simulink model "feedbackLinearizationMambo"  (R2021a)
settings: Solver=VariableStepAuto  StartTime=0.0  StopTime=10  FixedStep=4e-3  RelTol=1e-12
InitFcn:
  | init
values from neighbouring files (symbols this model uses):
  a = 4.7200e-08*13840.8    (= 0.00065328576)    [init.m]
  c = 1.1393e-10*13840.8    (= 1.576882344e-06)    [init.m]
  g = 9.31    [init.m]
  isMambo = true    [init.m]
  J = [Jx;Jy;Jz]    [init.m]
  Jx = 5.82857e-5    (= 5.82857e-05)    [init.m]
  Jy = 7.169148e-5    (= 7.169148e-05)    [init.m]
  Jz = 1e-4    (= 0.0001)    [init.m]
  Ki = [0.1 0.6 0.1]*0    [init.m]
  Kp = [0.6 0.7 1]*50    [init.m]
  Kw = [0.08 0.1 0.2]*100    [init.m]
  l = 0.0624*2    (= 0.1248)    [init.m]
  m = 0.063    [init.m]
  posNED = [57 95 -0.046]    [init.m]
  sigma = [l*a/Jx l*a/Jy l*a/Jz a/m]    [init.m]
  T = 0.0050    (= 0.005)    [init.m]
undefined symbols (not defined in the file or in its folder): DiscIntNeverNeededParam, Earth, init, rho, Vehicle, WGS84
libraries: pid_lib x14, sharedtransform x6, simulink x2, shared6dof x1, aerolibasang x1, aerolibtransform2 x1, vrlib x1
(part 1 of 2)
settings Model: Creator=dbnun  LastModifiedBy=dbnun
settings SolverCC: AlgebraicLoopSolver=TrustRegion

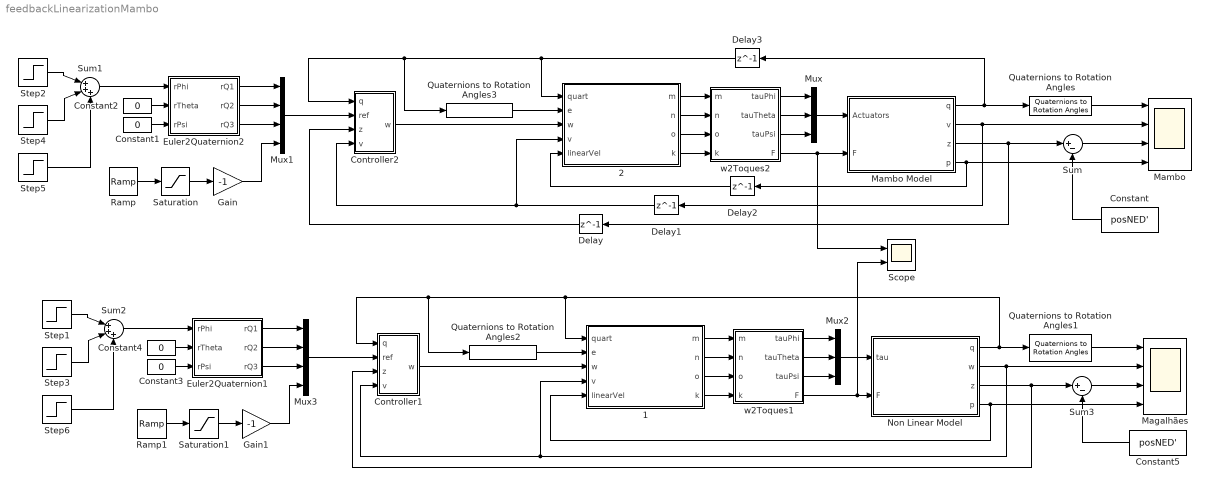
== system feedbackLinearizationMambo ==
  " 1" : MATLAB Function  TreatAsAtomicUnit=on
  " 2" : MATLAB Function  TreatAsAtomicUnit=on
  Constant : Constant  Value=posNED'
  Constant{1..4} (4 alike) : Constant  Value=0
  Constant5 : Constant  Value=posNED'
  Controller1 : Subsystem
  Controller2 : Subsystem
  Delay : Delay  DelayLength=1  InitialCondition=posNED'
  Delay1 : Delay  DelayLength=1
  Delay2 : Delay  DelayLength=1
  Delay3 : Delay  DelayLength=1  InitialCondition=[1 0 0 0]
  Euler2Quaternion1 : Subsystem
  Euler2Quaternion2 : Subsystem
  Gain : Gain  Gain=-1
  Gain1 : Gain  Gain=-1
  Magalhães : Scope  NumInputPorts=4
  Mambo : Scope  NumInputPorts=4
  Mambo Model : Subsystem
  Mux : Mux  Inputs=3
  Mux1 : Mux
  Mux2 : Mux  Inputs=3
  Mux3 : Mux
  Non Linear Model : Subsystem
  Quaternions to Rotation Angles{,1..3} (4 alike) : sharedtransform/Quaternions to Rotation Angles  rotationOrder=XYZ  aMode=aMode
      settings: SourceProductBaseCode=AE,PW,DR,MT,UV,VE
  Ramp : simulink/Sources/Ramp  slope=2  start=0  InitialOutput=0
  Ramp1 : simulink/Sources/Ramp  slope=2  start=0  InitialOutput=0
  Saturation : Saturate  UpperLimit=1  LowerLimit=0
  Saturation1 : Saturate  UpperLimit=1  LowerLimit=0
  Scope : Scope  NumInputPorts=2
  Step1 : Step  Time=2  After=2*pi/180  SampleTime=0
  Step2 : Step  Time=2  After=2*pi/180  SampleTime=0
  Step3 : Step  Time=3  After=-3*pi/180  SampleTime=0
  Step4 : Step  Time=3  After=-3*pi/180  SampleTime=0
  Step5 : Step  Time=3.5  After=1*pi/180  SampleTime=0
  Step6 : Step  Time=3.5  After=1*pi/180  SampleTime=0
  Sum : Sum  Inputs=|+-
  Sum1 : Sum  Inputs=|+++
  Sum2 : Sum  Inputs=|+++
  Sum3 : Sum  Inputs=|+-
  w2Toques1 : Subsystem
  w2Toques2 : Subsystem
  wires:
  Mux/1 -> Mambo Model/1(Actuators)
  w2Toques2/1(tauPhi) -> Mux/1
  w2Toques2/2(tauTheta) -> Mux/2
  w2Toques2/3(tauPsi) -> Mux/3
  Quaternions to Rotation Angles/1 -> Mambo/1
  Quaternions to Rotation Angles1/1 -> Magalhães/1
  w2Toques1/3(tauPsi) -> Mux2/3
  Mux3/1 -> Controller1/2(ref)
  Non Linear Model/1(q) -> Quaternions to Rotation Angles2/1, Controller1/1(q), " 1"/1(quart), Quaternions to Rotation Angles1/1
  w2Toques1/1(tauPhi) -> Mux2/1
  " 1"/3(o) -> w2Toques1/3(o)
  Euler2Quaternion1/1(rQ1) -> Mux3/1
  " 1"/1(m) -> w2Toques1/1(m)
  Non Linear Model/2(w) -> Magalhães/2, " 1"/4(v), Controller1/4(v)
  " 1"/2(n) -> w2Toques1/2(n)
  w2Toques1/2(tauTheta) -> Mux2/2
  Euler2Quaternion1/2(rQ2) -> Mux3/2
  Euler2Quaternion1/3(rQ3) -> Mux3/3
  " 1"/4(k) -> w2Toques1/4(k)
  Non Linear Model/4(p) -> Magalhães/4, " 1"/5(linearVel)
  Non Linear Model/3(z) -> Sum3/1, Controller1/3(z)
  Mux2/1 -> Non Linear Model/1(tau)
  Controller1/1(w) -> " 1"/3(w)
  Quaternions to Rotation Angles2/1 -> " 1"/2(e)
  Constant1/1 -> Euler2Quaternion2/3(rPsi)
  Constant2/1 -> Euler2Quaternion2/2(rTheta)
  Controller2/1(w) -> " 2"/3(w)
  Euler2Quaternion2/2(rQ2) -> Mux1/2
  " 2"/2(n) -> w2Toques2/2(n)
  " 2"/3(o) -> w2Toques2/3(o)
  Euler2Quaternion2/1(rQ1) -> Mux1/1
  Mambo Model/2(v) -> Delay1/1, Mambo/2
  Mambo Model/1(q) -> Delay3/1, Quaternions to Rotation Angles/1
  Mambo Model/4(p) -> Mambo/4, Delay2/1
  Sum1/1 -> Euler2Quaternion2/1(rPhi)
  Mux1/1 -> Controller2/2(ref)
  Step5/1 -> Sum1/3
  Step4/1 -> Sum1/2
  " 2"/1(m) -> w2Toques2/1(m)
  Quaternions to Rotation Angles3/1 -> " 2"/2(e)
  Euler2Quaternion2/3(rQ3) -> Mux1/3
  Step2/1 -> Sum1/1
  Mambo Model/3(z) -> Sum/1, Delay/1
  w2Toques2/4(F) -> Scope/1, Mambo Model/2(F)
  " 2"/4(k) -> w2Toques2/4(k)
  Delay/1 -> Controller2/3(z)
  Delay1/1 -> " 2"/4(v), Controller2/4(v)
  Delay2/1 -> " 2"/5(linearVel)
  Delay3/1 -> " 2"/1(quart), Controller2/1(q), Quaternions to Rotation Angles3/1
  w2Toques1/4(F) -> Scope/2, Non Linear Model/2(F)
  Step6/1 -> Sum2/3
  Sum2/1 -> Euler2Quaternion1/1(rPhi)
  Step3/1 -> Sum2/2
  Step1/1 -> Sum2/1
  Constant4/1 -> Euler2Quaternion1/2(rTheta)
  Constant3/1 -> Euler2Quaternion1/3(rPsi)
  Sum/1 -> Mambo/3
  Sum3/1 -> Magalhães/3
  Constant/1 -> Sum/2
  Constant5/1 -> Sum3/2
  Saturation/1 -> Gain/1
  Ramp/1 -> Saturation/1
  Gain/1 -> Mux1/4
  Gain1/1 -> Mux3/4
  Saturation1/1 -> Gain1/1
  Ramp1/1 -> Saturation1/1

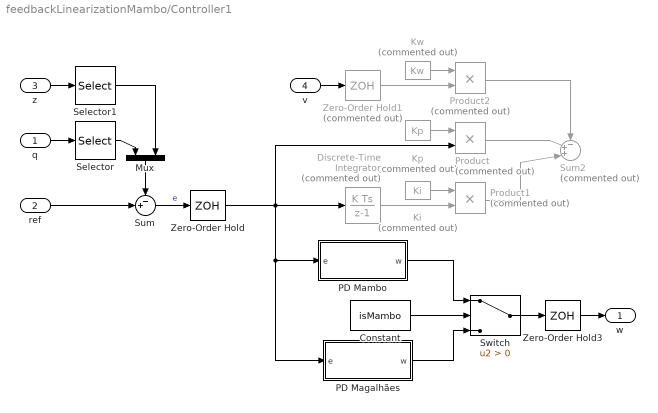
== system feedbackLinearizationMambo/Controller1 ==
  q : Inport
  ref : Inport  Port=2
  z : Inport  Port=3
  v : Inport  Port=4
  Constant : Constant  Value=isMambo
  Discrete-Time Integrator : DiscreteIntegrator  Commented=on  SampleTime=T  ICPrevOutput=DiscIntNeverNeededParam  ICPrevScaledInput=DiscIntNeverNeededParam
  Ki : Constant  Commented=on  Value=Ki
  Kp : Constant  Commented=on  Value=Kp
  Kw : Constant  Commented=on  Value=Kw  VectorParams1D=off
  Mux : Mux  Inputs=2
  PD Magalhães : Subsystem
  PD Mambo : Subsystem
  Product : Product  Commented=on
  Product1 : Product  Commented=on
  Product2 : Product  Commented=on
  Selector : Selector  InputPortWidth=4  IndexOptions=Index vector (dialog)  Indices=[2 3 4]  OutputSizes=1
  Selector1 : Selector  InputPortWidth=3  IndexOptions=Index vector (dialog)  Indices=[3]  OutputSizes=1
  Sum : Sum  Inputs=-+|
  Sum2 : Sum  Commented=on  Inputs=-++|
  Switch : Switch  Criteria=u2 > Threshold
  Zero-Order Hold : ZeroOrderHold  SampleTime=T
  Zero-Order Hold1 : ZeroOrderHold  Commented=on  SampleTime=T
  Zero-Order Hold3 : ZeroOrderHold  SampleTime=T
  w : Outport
  wires:
  Ki/1 -> Product1/1
  Selector/1 -> Mux/1
  q/1 -> Selector/1
  Product1/1 -> Sum2/3
  Sum/1 -> Zero-Order Hold/1  "e"
  ref/1 -> Sum/2
  Kw/1 -> Product2/1
  Product/1 -> Sum2/2
  Product2/1 -> Sum2/1
  Kp/1 -> Product/1
  v/1 -> Zero-Order Hold1/1
  Discrete-Time Integrator/1 -> Product1/2
  Zero-Order Hold/1 -> PD Magalhães/1(e), PD Mambo/1(e), Product/2, Discrete-Time Integrator/1
  Zero-Order Hold1/1 -> Product2/2
  PD Mambo/1(w) -> Switch/1
  Constant/1 -> Switch/2
  PD Magalhães/1(w) -> Switch/3
  Switch/1 -> Zero-Order Hold3/1
  Zero-Order Hold3/1 -> w/1
  z/1 -> Selector1/1
  Mux/1 -> Sum/1
  Selector1/1 -> Mux/2

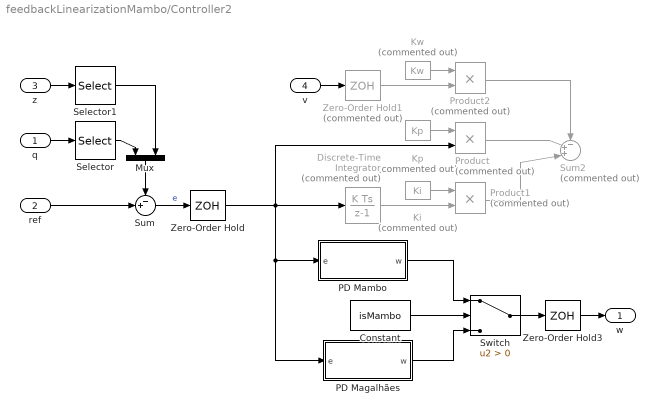
== system feedbackLinearizationMambo/Controller2 ==
  q : Inport
  ref : Inport  Port=2
  z : Inport  Port=3
  v : Inport  Port=4
  Constant : Constant  Value=isMambo
  Discrete-Time Integrator : DiscreteIntegrator  Commented=on  SampleTime=T  ICPrevOutput=DiscIntNeverNeededParam  ICPrevScaledInput=DiscIntNeverNeededParam
  Ki : Constant  Commented=on  Value=Ki
  Kp : Constant  Commented=on  Value=Kp
  Kw : Constant  Commented=on  Value=Kw  VectorParams1D=off
  Mux : Mux  Inputs=2
  PD Magalhães : Subsystem
  PD Mambo : Subsystem
  Product : Product  Commented=on
  Product1 : Product  Commented=on
  Product2 : Product  Commented=on
  Selector : Selector  InputPortWidth=4  IndexOptions=Index vector (dialog)  Indices=[2 3 4]  OutputSizes=1
  Selector1 : Selector  InputPortWidth=3  IndexOptions=Index vector (dialog)  Indices=[3]  OutputSizes=1
  Sum : Sum  Inputs=-+|
  Sum2 : Sum  Commented=on  Inputs=-++|
  Switch : Switch  Criteria=u2 > Threshold
  Zero-Order Hold : ZeroOrderHold  SampleTime=T
  Zero-Order Hold1 : ZeroOrderHold  Commented=on  SampleTime=T
  Zero-Order Hold3 : ZeroOrderHold  SampleTime=T
  w : Outport
  wires:
  Ki/1 -> Product1/1
  Selector/1 -> Mux/1
  q/1 -> Selector/1
  Product1/1 -> Sum2/3
  Sum/1 -> Zero-Order Hold/1  "e"
  ref/1 -> Sum/2
  Kw/1 -> Product2/1
  Product/1 -> Sum2/2
  Product2/1 -> Sum2/1
  Kp/1 -> Product/1
  v/1 -> Zero-Order Hold1/1
  Discrete-Time Integrator/1 -> Product1/2
  Zero-Order Hold/1 -> PD Magalhães/1(e), PD Mambo/1(e), Product/2, Discrete-Time Integrator/1
  Zero-Order Hold1/1 -> Product2/2
  PD Mambo/1(w) -> Switch/1
  Constant/1 -> Switch/2
  PD Magalhães/1(w) -> Switch/3
  Switch/1 -> Zero-Order Hold3/1
  Zero-Order Hold3/1 -> w/1
  z/1 -> Selector1/1
  Mux/1 -> Sum/1
  Selector1/1 -> Mux/2

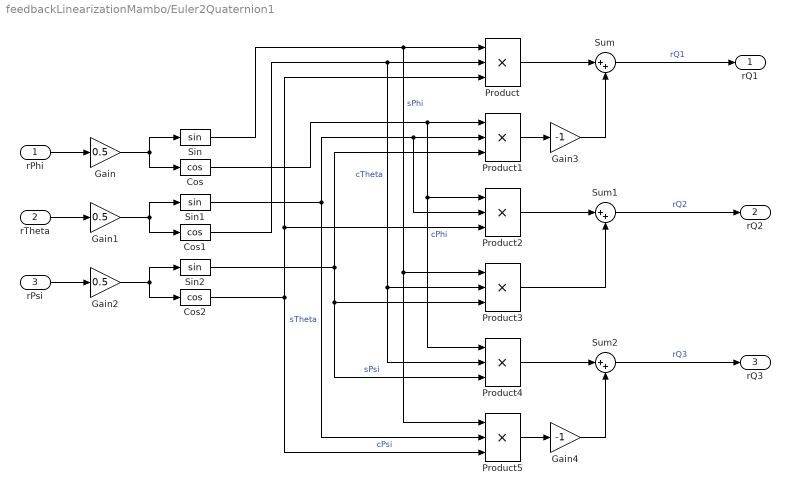
== system feedbackLinearizationMambo/Euler2Quaternion1 ==
  rPhi : Inport
  rTheta : Inport  Port=2
  rPsi : Inport  Port=3
  Cos : Trigonometry  Operator=cos
  Cos1 : Trigonometry  Operator=cos
  Cos2 : Trigonometry  Operator=cos
  Gain : Gain  Gain=0.5
  Gain1 : Gain  Gain=0.5
  Gain2 : Gain  Gain=0.5
  Gain3 : Gain  Gain=-1
  Gain4 : Gain  Gain=-1
  Product{,1..5} (6 alike) : Product  Inputs=3
  Sin : Trigonometry
  Sin1 : Trigonometry
  Sin2 : Trigonometry
  Sum : Sum  Inputs=|++
  Sum1 : Sum  Inputs=|++
  Sum2 : Sum  Inputs=|++
  rQ1 : Outport
  rQ2 : Outport  Port=2
  rQ3 : Outport  Port=3
  wires:
  Sum1/1 -> rQ2/1  "rQ2"
  rTheta/1 -> Gain1/1
  Gain/1 -> Sin/1, Cos/1
  rPsi/1 -> Gain2/1
  Sin1/1 -> Product2/2, Product1/2, Product5/2  "sTheta"
  Gain2/1 -> Sin2/1, Cos2/1
  rPhi/1 -> Gain/1
  Gain1/1 -> Sin1/1, Cos1/1
  Sin2/1 -> Product4/3, Product3/3, Product1/3  "sPsi"
  Cos/1 -> Product4/1, Product2/1, Product1/1  "cPhi"
  Sum2/1 -> rQ3/1  "rQ3"
  Cos2/1 -> Product2/3, Product/3, Product5/3  "cPsi"
  Sin/1 -> Product5/1, Product3/1, Product/1  "sPhi"
  Gain3/1 -> Sum/2
  Cos1/1 -> Product4/2, Product3/2, Product/2  "cTheta"
  Product1/1 -> Gain3/1
  Product/1 -> Sum/1
  Product5/1 -> Gain4/1
  Product3/1 -> Sum1/2
  Product2/1 -> Sum1/1
  Product4/1 -> Sum2/1
  Gain4/1 -> Sum2/2
  Sum/1 -> rQ1/1  "rQ1"

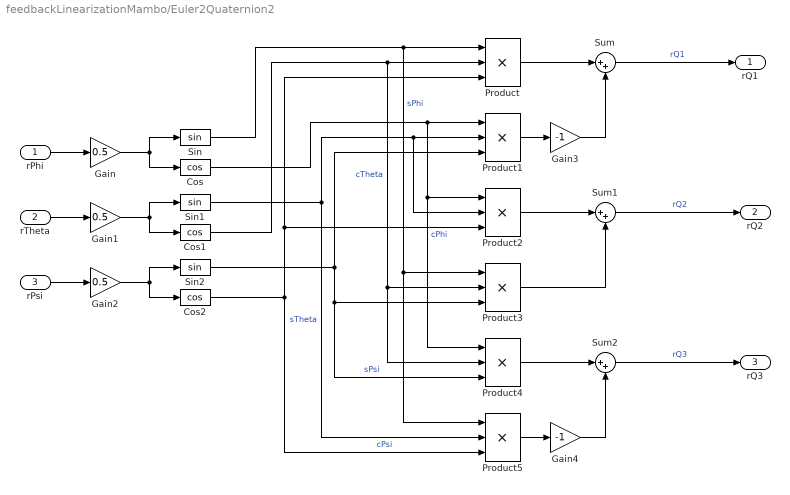
== system feedbackLinearizationMambo/Euler2Quaternion2 ==
  rPhi : Inport
  rTheta : Inport  Port=2
  rPsi : Inport  Port=3
  Cos : Trigonometry  Operator=cos
  Cos1 : Trigonometry  Operator=cos
  Cos2 : Trigonometry  Operator=cos
  Gain : Gain  Gain=0.5
  Gain1 : Gain  Gain=0.5
  Gain2 : Gain  Gain=0.5
  Gain3 : Gain  Gain=-1
  Gain4 : Gain  Gain=-1
  Product{,1..5} (6 alike) : Product  Inputs=3
  Sin : Trigonometry
  Sin1 : Trigonometry
  Sin2 : Trigonometry
  Sum : Sum  Inputs=|++
  Sum1 : Sum  Inputs=|++
  Sum2 : Sum  Inputs=|++
  rQ1 : Outport
  rQ2 : Outport  Port=2
  rQ3 : Outport  Port=3
  wires:
  Sum1/1 -> rQ2/1  "rQ2"
  rTheta/1 -> Gain1/1
  Gain/1 -> Sin/1, Cos/1
  rPsi/1 -> Gain2/1
  Sin1/1 -> Product2/2, Product1/2, Product5/2  "sTheta"
  Gain2/1 -> Sin2/1, Cos2/1
  rPhi/1 -> Gain/1
  Gain1/1 -> Sin1/1, Cos1/1
  Sin2/1 -> Product4/3, Product3/3, Product1/3  "sPsi"
  Cos/1 -> Product4/1, Product2/1, Product1/1  "cPhi"
  Sum2/1 -> rQ3/1  "rQ3"
  Cos2/1 -> Product2/3, Product/3, Product5/3  "cPsi"
  Sin/1 -> Product5/1, Product3/1, Product/1  "sPhi"
  Gain3/1 -> Sum/2
  Cos1/1 -> Product4/2, Product3/2, Product/2  "cTheta"
  Product1/1 -> Gain3/1
  Product/1 -> Sum/1
  Product5/1 -> Gain4/1
  Product3/1 -> Sum1/2
  Product2/1 -> Sum1/1
  Product4/1 -> Sum2/1
  Gain4/1 -> Sum2/2
  Sum/1 -> rQ1/1  "rQ1"

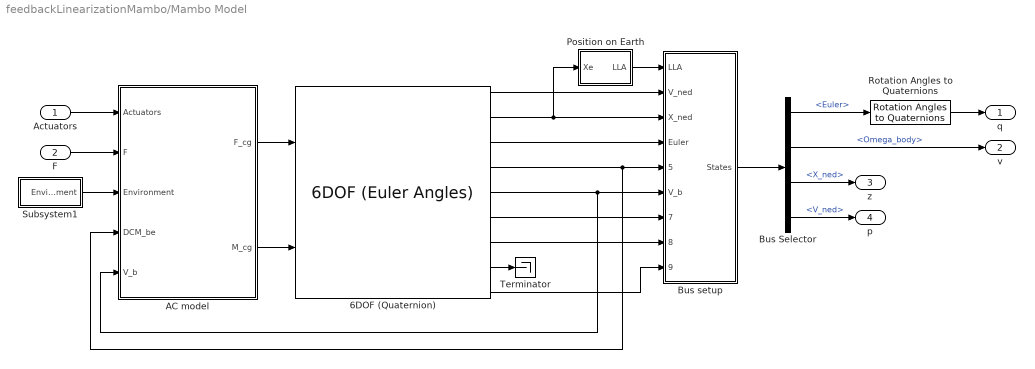
== system feedbackLinearizationMambo/Mambo Model ==
  Actuators : Inport
  F : Inport  Port=2
  6DOF (Quaternion) : shared6dof/6DOF (Euler Angles)  units=Metric (MKS)  mtype=Fixed  rep=Euler Angles  xme_0=init.posNED  Vm_0=init.vb  eul_0=init.euler  pm_0=init.angRates  mass_0=Vehicle.Airframe.mass  mass_e=0.5  mass_f=2.0  inertia=Vehicle.Airframe.inertia  inertia_e=eye(3)  inertia_f=2*eye(3)  k_quat=Vehicle.SixDOF.quatGain  vre_flag=on  abi_flag=on  aMode=aMode  xme_statename=''  Vm_statename=''  eul_statename=''  quat_statename=''  pm_statename=''  mass_statename=''
      settings: SourceProductBaseCode=AE,PW,DR,MT,UV,VE
  AC model : Subsystem
  Bus Selector : BusSelector  OutputSignals=Euler,Omega_body,X_ned,V_ned
  Bus setup : Subsystem
  Position on Earth : Subsystem  Priority=1  TreatAsAtomicUnit=on
  Rotation Angles to Quaternions : sharedtransform/Rotation Angles to Quaternions  rotationOrder=XYZ  aMode=aMode
      settings: SourceProductBaseCode=AE,PW,DR,MT,UV,VE
  Subsystem1 : Subsystem
  Terminator : Terminator
  q : Outport
  v : Outport  Port=2
  z : Outport  Port=3
  p : Outport  Port=4
  wires:
  Position on Earth/1(LLA) -> Bus setup/1(LLA)
  6DOF (Quaternion)/5 -> AC model/5(V_b), Bus setup/6(V_b)
  6DOF (Quaternion)/7 -> Bus setup/8(dOmega_b)
  Subsystem1/1(Environment) -> AC model/3(Environment)
  6DOF (Quaternion)/1 -> Bus setup/2(V_ned)
  6DOF (Quaternion)/8 -> Terminator/1
  Bus setup/1(States) -> Bus Selector/1
  AC model/1(F_cg) -> 6DOF (Quaternion)/1
  6DOF (Quaternion)/6 -> Bus setup/7(Omega_b)
  6DOF (Quaternion)/2 -> Position on Earth/1(Xe), Bus setup/3(X_ned)
  6DOF (Quaternion)/3 -> Bus setup/4(Euler)
  Actuators/1 -> AC model/1(Actuators)
  6DOF (Quaternion)/9 -> Bus setup/9(Accel_b)
  AC model/2(M_cg) -> 6DOF (Quaternion)/2
  6DOF (Quaternion)/4 -> AC model/4(DCM_be), Bus setup/5(DCM_be)
  Bus Selector/1 -> Rotation Angles to Quaternions/1  "<Euler>"
  Rotation Angles to Quaternions/1 -> q/1
  Bus Selector/2 -> v/1  "<Omega_body>"
  Bus Selector/3 -> z/1  "<X_ned>"
  Bus Selector/4 -> p/1  "<V_ned>"
  F/1 -> AC model/2(F)

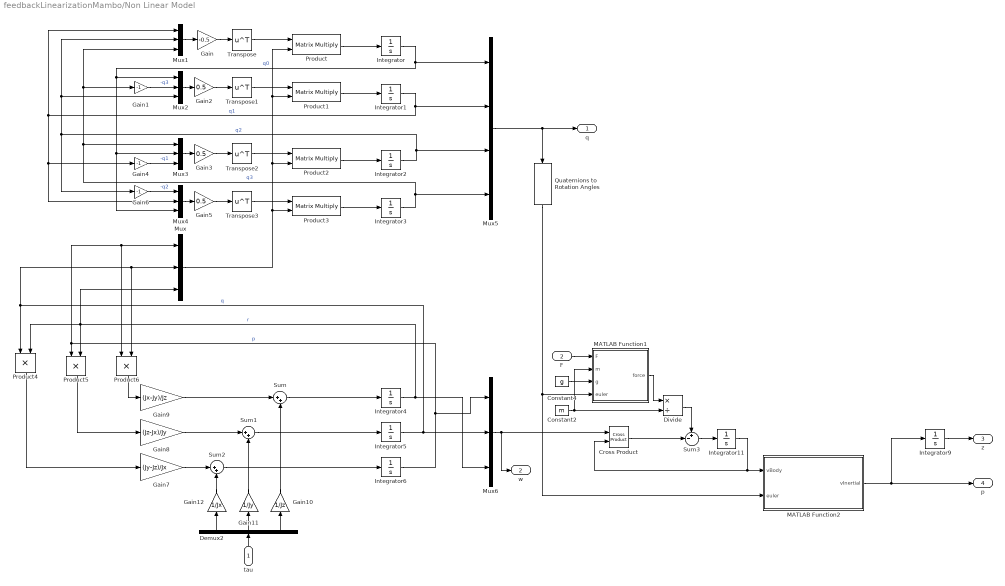
== system feedbackLinearizationMambo/Non Linear Model ==
  tau : Inport
  F : Inport  Port=2
  Constant2 : Constant  Value=m
  Constant4 : Constant  Value=g
  Cross Product : vrlib/Utilities/Cross Product
  Demux2 : Demux  Outputs=3
  Divide : Product  Inputs=*/
  Gain : Gain  Gain=-0.5
  Gain1 : Gain  Gain=-1
  Gain10 : Gain  Gain=1/Jz
  Gain11 : Gain  Gain=1/Jy
  Gain12 : Gain  Gain=1/Jx
  Gain2 : Gain  Gain=0.5
  Gain3 : Gain  Gain=0.5
  Gain4 : Gain  Gain=-1
  Gain5 : Gain  Gain=0.5
  Gain6 : Gain  Gain=-1
  Gain7 : Gain  Gain=(Jy-Jz)/Jx
  Gain8 : Gain  Gain=(Jz-Jx)/Jy
  Gain9 : Gain  Gain=(Jx-Jy)/Jz
  Integrator : Integrator  InitialCondition=1
  Integrator{1..6} (6 alike) : Integrator
  Integrator11 : Integrator  InitialCondition=[0 0 0]
  Integrator9 : Integrator  InitialCondition=posNED
  MATLAB Function1 : MATLAB Function  TreatAsAtomicUnit=on
  MATLAB Function2 : MATLAB Function  TreatAsAtomicUnit=on
  Mux{,1..4,6} (6 alike) : Mux  Inputs=3
  Mux5 : Mux
  Product{,1..3} (4 alike) : Product  Multiplication=Matrix(*)
  Product4 : Product
  Product5 : Product
  Product6 : Product
  Quaternions to Rotation Angles : sharedtransform/Quaternions to Rotation Angles  rotationOrder=XYZ  aMode=aMode
      settings: SourceProductBaseCode=AE,PW,DR,MT,UV,VE
  Sum : Sum  Inputs=|++
  Sum1 : Sum  Inputs=|++
  Sum2 : Sum  Inputs=|++
  Sum3 : Sum  Inputs=+-|
  Transpose{,1..3} (4 alike) : Math  Operator=transpose  SaturateOnIntegerOverflow=on
  q : Outport
  w : Outport  Port=2
  z : Outport  Port=3
  p : Outport  Port=4
  wires:
  Product1/1 -> Integrator1/1
  Gain4/1 -> Mux3/3  "-q1"
  Gain6/1 -> Mux4/1  "-q2"
  Integrator4/1 -> Product5/2, Product4/2, Mux/3, Mux6/3  "r"
  Integrator3/1 -> Mux3/1, Mux1/3, Gain1/1, Mux5/4  "q3"
  Integrator/1 -> Mux4/3, Mux3/2, Mux2/1, Mux5/1  "q0"
  Gain1/1 -> Mux2/2  "-q3"
  Gain/1 -> Transpose/1
  Transpose3/1 -> Product3/1
  Sum2/1 -> Integrator6/1
  Mux2/1 -> Gain2/1
  Product4/1 -> Gain7/1
  Integrator5/1 -> Product6/2, Mux/2, Product4/1, Mux6/2  "q"
  Transpose1/1 -> Product1/1
  Integrator1/1 -> Mux1/1, Gain4/1, Mux4/2, Mux5/2  "q1"
  Integrator2/1 -> Mux2/3, Mux1/2, Gain6/1, Mux5/3  "q2"
  Mux/1 -> Product/2, Product1/2, Product2/2, Product3/2
  Mux4/1 -> Gain5/1
  Integrator6/1 -> Product5/1, Product6/1, Mux/1, Mux6/1  "p"
  Gain5/1 -> Transpose3/1
  Mux1/1 -> Gain/1
  Gain2/1 -> Transpose1/1
  Transpose/1 -> Product/1
  Product2/1 -> Integrator2/1
  Mux3/1 -> Gain3/1
  Transpose2/1 -> Product2/1
  Sum/1 -> Integrator4/1
  Product6/1 -> Gain9/1
  Product3/1 -> Integrator3/1
  Gain3/1 -> Transpose2/1
  Product/1 -> Integrator/1
  Product5/1 -> Gain8/1
  Sum1/1 -> Integrator5/1
  tau/1 -> Demux2/1
  Mux5/1 -> q/1, Quaternions to Rotation Angles/1
  Gain9/1 -> Sum/1
  Gain8/1 -> Sum1/1
  Gain7/1 -> Sum2/1
  Gain10/1 -> Sum/2
  Gain11/1 -> Sum1/2
  Gain12/1 -> Sum2/2
  Demux2/1 -> Gain12/1
  Demux2/2 -> Gain11/1
  Demux2/3 -> Gain10/1
  Constant2/1 -> MATLAB Function1/2(m), Divide/2
  Divide/1 -> Sum3/1
  Cross Product/1 -> Sum3/2
  Mux6/1 -> Cross Product/1, w/1
  Sum3/1 -> Integrator11/1
  Constant4/1 -> MATLAB Function1/3(g)
  Integrator11/1 -> MATLAB Function2/1(vBody), Cross Product/2
  Quaternions to Rotation Angles/1 -> MATLAB Function1/4(euler), MATLAB Function2/2(euler)
  Integrator9/1 -> z/1
  MATLAB Function2/1(vInertial) -> Integrator9/1, p/1
  MATLAB Function1/1(force) -> Divide/1
  F/1 -> MATLAB Function1/1(F)

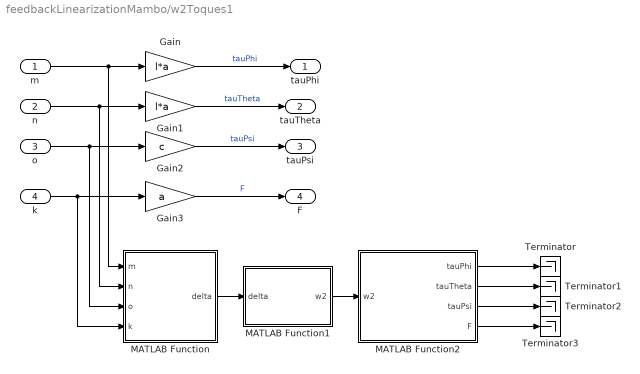
== system feedbackLinearizationMambo/w2Toques1 ==
  m : Inport
  n : Inport  Port=2
  o : Inport  Port=3
  k : Inport  Port=4
  Gain : Gain  Gain=l*a
  Gain1 : Gain  Gain=l*a
  Gain2 : Gain  Gain=c
  Gain3 : Gain  Gain=a
  MATLAB Function : MATLAB Function  TreatAsAtomicUnit=on
  MATLAB Function1 : MATLAB Function  TreatAsAtomicUnit=on
  MATLAB Function2 : MATLAB Function  TreatAsAtomicUnit=on
  Terminator{,1..3} (4 alike) : Terminator
  tauPhi : Outport
  tauTheta : Outport  Port=2
  tauPsi : Outport  Port=3
  F : Outport  Port=4
  wires:
  Gain/1 -> tauPhi/1  "tauPhi"
  o/1 -> MATLAB Function/3(o), Gain2/1
  n/1 -> MATLAB Function/2(n), Gain1/1
  Gain1/1 -> tauTheta/1  "tauTheta"
  m/1 -> MATLAB Function/1(m), Gain/1
  Gain2/1 -> tauPsi/1  "tauPsi"
  Gain3/1 -> F/1  "F"
  k/1 -> MATLAB Function/4(k), Gain3/1
  MATLAB Function/1(delta) -> MATLAB Function1/1(delta)
  MATLAB Function1/1(w2) -> MATLAB Function2/1(w2)
  MATLAB Function2/1(tauPhi) -> Terminator/1
  MATLAB Function2/2(tauTheta) -> Terminator1/1
  MATLAB Function2/3(tauPsi) -> Terminator2/1
  MATLAB Function2/4(F) -> Terminator3/1

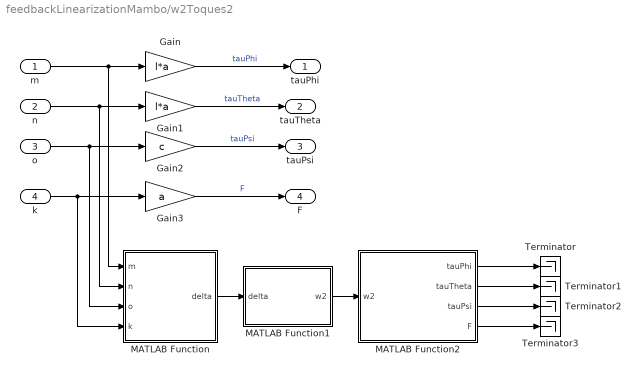
== system feedbackLinearizationMambo/w2Toques2 ==
  m : Inport
  n : Inport  Port=2
  o : Inport  Port=3
  k : Inport  Port=4
  Gain : Gain  Gain=l*a
  Gain1 : Gain  Gain=l*a
  Gain2 : Gain  Gain=c
  Gain3 : Gain  Gain=a
  MATLAB Function : MATLAB Function  TreatAsAtomicUnit=on
  MATLAB Function1 : MATLAB Function  TreatAsAtomicUnit=on
  MATLAB Function2 : MATLAB Function  TreatAsAtomicUnit=on
  Terminator{,1..3} (4 alike) : Terminator
  tauPhi : Outport
  tauTheta : Outport  Port=2
  tauPsi : Outport  Port=3
  F : Outport  Port=4
  wires:
  Gain/1 -> tauPhi/1  "tauPhi"
  o/1 -> MATLAB Function/3(o), Gain2/1
  n/1 -> MATLAB Function/2(n), Gain1/1
  Gain1/1 -> tauTheta/1  "tauTheta"
  m/1 -> MATLAB Function/1(m), Gain/1
  Gain2/1 -> tauPsi/1  "tauPsi"
  Gain3/1 -> F/1  "F"
  k/1 -> MATLAB Function/4(k), Gain3/1
  MATLAB Function/1(delta) -> MATLAB Function1/1(delta)
  MATLAB Function1/1(w2) -> MATLAB Function2/1(w2)
  MATLAB Function2/1(tauPhi) -> Terminator/1
  MATLAB Function2/2(tauTheta) -> Terminator1/1
  MATLAB Function2/3(tauPsi) -> Terminator2/1
  MATLAB Function2/4(F) -> Terminator3/1

== system feedbackLinearizationMambo/Controller1/PD Magalhães ==
  e : Inport
  Demux1 : Demux  Outputs=3
  Discrete PID Controller3 : pid_lib/PID Controller  Controller=PD  Form=Parallel  TimeDomain=Discrete-time  UseExternalTs=off  SampleTime=T  IntegratorMethod=Forward Euler  FilterMethod=Forward Euler  ControllerParametersSource=internal  P=0.0004  I=Ki  D=0.0075  UseFilter=off  N=100  TunerSelectOption=Transfer Function Based (PID Tuner App)  InitialConditionSource=internal  InitialConditionForIntegrator=0  InitialConditionForFilter=0  DifferentiatorICPrevScaledInput=0  ExternalReset=none  TrackingMode=off  Kt=1  LimitOutput=off  SatLimitsSource=internal  UpperSaturationLimit=inf  LowerSaturationLimit=-inf  LinearizeAsGain=off  AntiWindupMode=none  Kb=1  POutMin=[]  POutMax=[]  IOutMin=[]  IOutMax=[]  DOutMin=[]  DOutMax=[]  NOutMin=[]  NOutMax=[]  SumOutMin=[]  SumOutMax=[]  SaturationOutMin=[]  SaturationOutMax=[]  PParamMin=[]  PParamMax=[]  IParamMin=[]  IParamMax=[]  DParamMin=[]  DParamMax=[]  NParamMin=[]  NParamMax=[]  KbParamMin=[]  KbParamMax=[]  KtParamMin=[]  KtParamMax=[]  KbOutMin=[]  KbOutMax=[]  KtOutMin=[]  KtOutMax=[]  IntegratorOutMin=[]  IntegratorOutMax=[]  FilterOutMin=[]  FilterOutMax=[]  SumI1OutMin=[]  SumI1OutMax=[]  SumI2OutMin=[]  SumI2OutMax=[]  SumI3OutMin=[]  SumI3OutMax=[]  SumI4OutMin=[]  SumI4OutMax=[]  SumDOutMin=[]  SumDOutMax=[]  DifferentiatorOutMin=[]  DifferentiatorOutMax=[]  FilterDiffOutCoefMin=[]  FilterDiffOutCoefMax=[]  ReciprocalOutMin=[]  ReciprocalOutMax=[]  SumDenOutMin=[]  SumDenOutMax=[]  SumNumOutMin=[]  SumNumOutMax=[]  DivideOutMin=[]  DivideOutMax=[]  UdiffTsProdOutMin=[]  UdiffTsProdOutMax=[]  NTsProdOutMin=[]  NTsProdOutMax=[]  UintegralTsProdOutMin=[]  UintegralTsProdOutMax=[]  UngainTsProdOutMin=[]  UngainTsProdOutMax=[]  IntegratorContinuousStateAttributes=''  IntegratorStateMustResolveToSignalObject=off  IntegratorRTWStateStorageClass=Auto  FilterContinuousStateAttributes=''  FilterStateMustResolveToSignalObject=off  FilterRTWStateStorageClass=Auto  ParallelPVariant=InternalParameters  IdealPVariant=Disabled  IVariant=Disabled  DVariant=InternalParameters  IntegratorVariant=Disabled  SatVariant=Disabled  AWVariant=Disabled  PCopyVariant=Disabled  TRVariant=Disabled  FdbkBlocksVariant=Forward  IdealPFdbkVariant=Disabled  SatFdbkVariant=Disabled  DerivativeFilterVariant=Differentiator  NVariant=Passthrough  NCopyVariant=Disabled_SignalSpec  FilterICVariant=InternalICsDifferentiator  IntegratorICVariant=Disabled  ExternalResetVariant=Disabled  TRSumVariant=Passthrough  SumFdbkVariant=Disabled  SumVariant=Sum_PD  TsampFilterVariant=InternalTs  TsampNgainVariant=Passthrough  TsampIntegralVariant=Disabled_SignalSpec  ExternalSaturationOutDataTypeStr=Inherit: Same as second input
  Discrete PID Controller4 : pid_lib/PID Controller  Controller=PD  Form=Parallel  TimeDomain=Discrete-time  UseExternalTs=off  SampleTime=T  IntegratorMethod=Forward Euler  FilterMethod=Forward Euler  ControllerParametersSource=internal  P=0.00025  I=Ki  D=0.0060  UseFilter=off  N=100  TunerSelectOption=Transfer Function Based (PID Tuner App)  InitialConditionSource=internal  InitialConditionForIntegrator=0  InitialConditionForFilter=0  DifferentiatorICPrevScaledInput=0  ExternalReset=none  TrackingMode=off  Kt=1  LimitOutput=off  SatLimitsSource=internal  UpperSaturationLimit=inf  LowerSaturationLimit=-inf  LinearizeAsGain=off  AntiWindupMode=none  Kb=1  POutMin=[]  POutMax=[]  IOutMin=[]  IOutMax=[]  DOutMin=[]  DOutMax=[]  NOutMin=[]  NOutMax=[]  SumOutMin=[]  SumOutMax=[]  SaturationOutMin=[]  SaturationOutMax=[]  PParamMin=[]  PParamMax=[]  IParamMin=[]  IParamMax=[]  DParamMin=[]  DParamMax=[]  NParamMin=[]  NParamMax=[]  KbParamMin=[]  KbParamMax=[]  KtParamMin=[]  KtParamMax=[]  KbOutMin=[]  KbOutMax=[]  KtOutMin=[]  KtOutMax=[]  IntegratorOutMin=[]  IntegratorOutMax=[]  FilterOutMin=[]  FilterOutMax=[]  SumI1OutMin=[]  SumI1OutMax=[]  SumI2OutMin=[]  SumI2OutMax=[]  SumI3OutMin=[]  SumI3OutMax=[]  SumI4OutMin=[]  SumI4OutMax=[]  SumDOutMin=[]  SumDOutMax=[]  DifferentiatorOutMin=[]  DifferentiatorOutMax=[]  FilterDiffOutCoefMin=[]  FilterDiffOutCoefMax=[]  ReciprocalOutMin=[]  ReciprocalOutMax=[]  SumDenOutMin=[]  SumDenOutMax=[]  SumNumOutMin=[]  SumNumOutMax=[]  DivideOutMin=[]  DivideOutMax=[]  UdiffTsProdOutMin=[]  UdiffTsProdOutMax=[]  NTsProdOutMin=[]  NTsProdOutMax=[]  UintegralTsProdOutMin=[]  UintegralTsProdOutMax=[]  UngainTsProdOutMin=[]  UngainTsProdOutMax=[]  IntegratorContinuousStateAttributes=''  IntegratorStateMustResolveToSignalObject=off  IntegratorRTWStateStorageClass=Auto  FilterContinuousStateAttributes=''  FilterStateMustResolveToSignalObject=off  FilterRTWStateStorageClass=Auto  ParallelPVariant=InternalParameters  IdealPVariant=Disabled  IVariant=Disabled  DVariant=InternalParameters  IntegratorVariant=Disabled  SatVariant=Disabled  AWVariant=Disabled  PCopyVariant=Disabled  TRVariant=Disabled  FdbkBlocksVariant=Forward  IdealPFdbkVariant=Disabled  SatFdbkVariant=Disabled  DerivativeFilterVariant=Differentiator  NVariant=Passthrough  NCopyVariant=Disabled_SignalSpec  FilterICVariant=InternalICsDifferentiator  IntegratorICVariant=Disabled  ExternalResetVariant=Disabled  TRSumVariant=Passthrough  SumFdbkVariant=Disabled  SumVariant=Sum_PD  TsampFilterVariant=InternalTs  TsampNgainVariant=Passthrough  TsampIntegralVariant=Disabled_SignalSpec  ExternalSaturationOutDataTypeStr=Inherit: Same as second input
  Discrete PID Controller5 : pid_lib/PID Controller  Controller=PD  Form=Parallel  TimeDomain=Discrete-time  UseExternalTs=off  SampleTime=T  IntegratorMethod=Forward Euler  FilterMethod=Forward Euler  ControllerParametersSource=internal  P=2e-05  I=Ki  D=0.00035  UseFilter=off  N=100  TunerSelectOption=Transfer Function Based (PID Tuner App)  InitialConditionSource=internal  InitialConditionForIntegrator=0  InitialConditionForFilter=0  DifferentiatorICPrevScaledInput=0  ExternalReset=none  TrackingMode=off  Kt=1  LimitOutput=off  SatLimitsSource=internal  UpperSaturationLimit=inf  LowerSaturationLimit=-inf  LinearizeAsGain=off  AntiWindupMode=none  Kb=1  POutMin=[]  POutMax=[]  IOutMin=[]  IOutMax=[]  DOutMin=[]  DOutMax=[]  NOutMin=[]  NOutMax=[]  SumOutMin=[]  SumOutMax=[]  SaturationOutMin=[]  SaturationOutMax=[]  PParamMin=[]  PParamMax=[]  IParamMin=[]  IParamMax=[]  DParamMin=[]  DParamMax=[]  NParamMin=[]  NParamMax=[]  KbParamMin=[]  KbParamMax=[]  KtParamMin=[]  KtParamMax=[]  KbOutMin=[]  KbOutMax=[]  KtOutMin=[]  KtOutMax=[]  IntegratorOutMin=[]  IntegratorOutMax=[]  FilterOutMin=[]  FilterOutMax=[]  SumI1OutMin=[]  SumI1OutMax=[]  SumI2OutMin=[]  SumI2OutMax=[]  SumI3OutMin=[]  SumI3OutMax=[]  SumI4OutMin=[]  SumI4OutMax=[]  SumDOutMin=[]  SumDOutMax=[]  DifferentiatorOutMin=[]  DifferentiatorOutMax=[]  FilterDiffOutCoefMin=[]  FilterDiffOutCoefMax=[]  ReciprocalOutMin=[]  ReciprocalOutMax=[]  SumDenOutMin=[]  SumDenOutMax=[]  SumNumOutMin=[]  SumNumOutMax=[]  DivideOutMin=[]  DivideOutMax=[]  UdiffTsProdOutMin=[]  UdiffTsProdOutMax=[]  NTsProdOutMin=[]  NTsProdOutMax=[]  UintegralTsProdOutMin=[]  UintegralTsProdOutMax=[]  UngainTsProdOutMin=[]  UngainTsProdOutMax=[]  IntegratorContinuousStateAttributes=''  IntegratorStateMustResolveToSignalObject=off  IntegratorRTWStateStorageClass=Auto  FilterContinuousStateAttributes=''  FilterStateMustResolveToSignalObject=off  FilterRTWStateStorageClass=Auto  ParallelPVariant=InternalParameters  IdealPVariant=Disabled  IVariant=Disabled  DVariant=InternalParameters  IntegratorVariant=Disabled  SatVariant=Disabled  AWVariant=Disabled  PCopyVariant=Disabled  TRVariant=Disabled  FdbkBlocksVariant=Forward  IdealPFdbkVariant=Disabled  SatFdbkVariant=Disabled  DerivativeFilterVariant=Differentiator  NVariant=Passthrough  NCopyVariant=Disabled_SignalSpec  FilterICVariant=InternalICsDifferentiator  IntegratorICVariant=Disabled  ExternalResetVariant=Disabled  TRSumVariant=Passthrough  SumFdbkVariant=Disabled  SumVariant=Sum_PD  TsampFilterVariant=InternalTs  TsampNgainVariant=Passthrough  TsampIntegralVariant=Disabled_SignalSpec  ExternalSaturationOutDataTypeStr=Inherit: Same as second input
  Mux1 : Mux  Inputs=3
  w : Outport
  wires:
  e/1 -> Demux1/1
  Discrete PID Controller3/1 -> Mux1/1
  Demux1/1 -> Discrete PID Controller3/1
  Demux1/3 -> Discrete PID Controller5/1
  Discrete PID Controller4/1 -> Mux1/2
  Discrete PID Controller5/1 -> Mux1/3
  Mux1/1 -> w/1
  Demux1/2 -> Discrete PID Controller4/1

== system feedbackLinearizationMambo/Controller1/PD Mambo ==
  e : Inport
  Demux : Demux
  Discrete PID Controller : pid_lib/PID Controller  Controller=PD  Form=Parallel  TimeDomain=Discrete-time  UseExternalTs=off  SampleTime=T  IntegratorMethod=Forward Euler  FilterMethod=Forward Euler  ControllerParametersSource=internal  P=0.625617124169113  I=Ki  D=7.14769061437549  UseFilter=on  N=296.310341187165  TunerSelectOption=Transfer Function Based (PID Tuner App)  InitialConditionSource=internal  InitialConditionForIntegrator=0  InitialConditionForFilter=0  DifferentiatorICPrevScaledInput=0  ExternalReset=none  TrackingMode=off  Kt=1  LimitOutput=off  SatLimitsSource=internal  UpperSaturationLimit=inf  LowerSaturationLimit=-inf  LinearizeAsGain=off  AntiWindupMode=none  Kb=1  POutMin=[]  POutMax=[]  IOutMin=[]  IOutMax=[]  DOutMin=[]  DOutMax=[]  NOutMin=[]  NOutMax=[]  SumOutMin=[]  SumOutMax=[]  SaturationOutMin=[]  SaturationOutMax=[]  PParamMin=[]  PParamMax=[]  IParamMin=[]  IParamMax=[]  DParamMin=[]  DParamMax=[]  NParamMin=[]  NParamMax=[]  KbParamMin=[]  KbParamMax=[]  KtParamMin=[]  KtParamMax=[]  KbOutMin=[]  KbOutMax=[]  KtOutMin=[]  KtOutMax=[]  IntegratorOutMin=[]  IntegratorOutMax=[]  FilterOutMin=[]  FilterOutMax=[]  SumI1OutMin=[]  SumI1OutMax=[]  SumI2OutMin=[]  SumI2OutMax=[]  SumI3OutMin=[]  SumI3OutMax=[]  SumI4OutMin=[]  SumI4OutMax=[]  SumDOutMin=[]  SumDOutMax=[]  DifferentiatorOutMin=[]  DifferentiatorOutMax=[]  FilterDiffOutCoefMin=[]  FilterDiffOutCoefMax=[]  ReciprocalOutMin=[]  ReciprocalOutMax=[]  SumDenOutMin=[]  SumDenOutMax=[]  SumNumOutMin=[]  SumNumOutMax=[]  DivideOutMin=[]  DivideOutMax=[]  UdiffTsProdOutMin=[]  UdiffTsProdOutMax=[]  NTsProdOutMin=[]  NTsProdOutMax=[]  UintegralTsProdOutMin=[]  UintegralTsProdOutMax=[]  UngainTsProdOutMin=[]  UngainTsProdOutMax=[]  IntegratorContinuousStateAttributes=''  IntegratorStateMustResolveToSignalObject=off  IntegratorRTWStateStorageClass=Auto  FilterContinuousStateAttributes=''  FilterStateMustResolveToSignalObject=off  FilterRTWStateStorageClass=Auto  ParallelPVariant=InternalParameters  IdealPVariant=Disabled  IVariant=Disabled  DVariant=InternalParameters  IntegratorVariant=Disabled  SatVariant=Disabled  AWVariant=Disabled  PCopyVariant=Disabled  TRVariant=Disabled  FdbkBlocksVariant=Forward  IdealPFdbkVariant=Disabled  SatFdbkVariant=Disabled  DerivativeFilterVariant=ForwardEulerFilter  NVariant=InternalParameters  NCopyVariant=Disabled  FilterICVariant=InternalICsFilter  IntegratorICVariant=Disabled  ExternalResetVariant=Disabled  TRSumVariant=Passthrough  SumFdbkVariant=Disabled  SumVariant=Sum_PD  TsampFilterVariant=InternalTs  TsampNgainVariant=Passthrough  TsampIntegralVariant=Disabled_SignalSpec  ExternalSaturationOutDataTypeStr=Inherit: Same as second input
  Discrete PID Controller1 : pid_lib/PID Controller  Controller=PD  Form=Parallel  TimeDomain=Discrete-time  UseExternalTs=off  SampleTime=T  IntegratorMethod=Forward Euler  FilterMethod=Forward Euler  ControllerParametersSource=internal  P=0.769509803348267  I=Ki  D=8.79166791728825  UseFilter=on  N=296.310341187165  TunerSelectOption=Transfer Function Based (PID Tuner App)  InitialConditionSource=internal  InitialConditionForIntegrator=0  InitialConditionForFilter=0  DifferentiatorICPrevScaledInput=0  ExternalReset=none  TrackingMode=off  Kt=1  LimitOutput=off  SatLimitsSource=internal  UpperSaturationLimit=inf  LowerSaturationLimit=-inf  LinearizeAsGain=off  AntiWindupMode=none  Kb=1  POutMin=[]  POutMax=[]  IOutMin=[]  IOutMax=[]  DOutMin=[]  DOutMax=[]  NOutMin=[]  NOutMax=[]  SumOutMin=[]  SumOutMax=[]  SaturationOutMin=[]  SaturationOutMax=[]  PParamMin=[]  PParamMax=[]  IParamMin=[]  IParamMax=[]  DParamMin=[]  DParamMax=[]  NParamMin=[]  NParamMax=[]  KbParamMin=[]  KbParamMax=[]  KtParamMin=[]  KtParamMax=[]  KbOutMin=[]  KbOutMax=[]  KtOutMin=[]  KtOutMax=[]  IntegratorOutMin=[]  IntegratorOutMax=[]  FilterOutMin=[]  FilterOutMax=[]  SumI1OutMin=[]  SumI1OutMax=[]  SumI2OutMin=[]  SumI2OutMax=[]  SumI3OutMin=[]  SumI3OutMax=[]  SumI4OutMin=[]  SumI4OutMax=[]  SumDOutMin=[]  SumDOutMax=[]  DifferentiatorOutMin=[]  DifferentiatorOutMax=[]  FilterDiffOutCoefMin=[]  FilterDiffOutCoefMax=[]  ReciprocalOutMin=[]  ReciprocalOutMax=[]  SumDenOutMin=[]  SumDenOutMax=[]  SumNumOutMin=[]  SumNumOutMax=[]  DivideOutMin=[]  DivideOutMax=[]  UdiffTsProdOutMin=[]  UdiffTsProdOutMax=[]  NTsProdOutMin=[]  NTsProdOutMax=[]  UintegralTsProdOutMin=[]  UintegralTsProdOutMax=[]  UngainTsProdOutMin=[]  UngainTsProdOutMax=[]  IntegratorContinuousStateAttributes=''  IntegratorStateMustResolveToSignalObject=off  IntegratorRTWStateStorageClass=Auto  FilterContinuousStateAttributes=''  FilterStateMustResolveToSignalObject=off  FilterRTWStateStorageClass=Auto  ParallelPVariant=InternalParameters  IdealPVariant=Disabled  IVariant=Disabled  DVariant=InternalParameters  IntegratorVariant=Disabled  SatVariant=Disabled  AWVariant=Disabled  PCopyVariant=Disabled  TRVariant=Disabled  FdbkBlocksVariant=Forward  IdealPFdbkVariant=Disabled  SatFdbkVariant=Disabled  DerivativeFilterVariant=ForwardEulerFilter  NVariant=InternalParameters  NCopyVariant=Disabled  FilterICVariant=InternalICsFilter  IntegratorICVariant=Disabled  ExternalResetVariant=Disabled  TRSumVariant=Passthrough  SumFdbkVariant=Disabled  SumVariant=Sum_PD  TsampFilterVariant=InternalTs  TsampNgainVariant=Passthrough  TsampIntegralVariant=Disabled_SignalSpec  ExternalSaturationOutDataTypeStr=Inherit: Same as second input
  Discrete PID Controller2 : pid_lib/PID Controller  Controller=PD  Form=Parallel  TimeDomain=Discrete-time  UseExternalTs=off  SampleTime=T  IntegratorMethod=Forward Euler  FilterMethod=Forward Euler  ControllerParametersSource=internal  P=130.980048513602  I=Ki  D=195.85931761802  UseFilter=on  N=189.861187655288  TunerSelectOption=Transfer Function Based (PID Tuner App)  InitialConditionSource=internal  InitialConditionForIntegrator=0  InitialConditionForFilter=0  DifferentiatorICPrevScaledInput=0  ExternalReset=none  TrackingMode=off  Kt=1  LimitOutput=off  SatLimitsSource=internal  UpperSaturationLimit=inf  LowerSaturationLimit=-inf  LinearizeAsGain=off  AntiWindupMode=none  Kb=1  POutMin=[]  POutMax=[]  IOutMin=[]  IOutMax=[]  DOutMin=[]  DOutMax=[]  NOutMin=[]  NOutMax=[]  SumOutMin=[]  SumOutMax=[]  SaturationOutMin=[]  SaturationOutMax=[]  PParamMin=[]  PParamMax=[]  IParamMin=[]  IParamMax=[]  DParamMin=[]  DParamMax=[]  NParamMin=[]  NParamMax=[]  KbParamMin=[]  KbParamMax=[]  KtParamMin=[]  KtParamMax=[]  KbOutMin=[]  KbOutMax=[]  KtOutMin=[]  KtOutMax=[]  IntegratorOutMin=[]  IntegratorOutMax=[]  FilterOutMin=[]  FilterOutMax=[]  SumI1OutMin=[]  SumI1OutMax=[]  SumI2OutMin=[]  SumI2OutMax=[]  SumI3OutMin=[]  SumI3OutMax=[]  SumI4OutMin=[]  SumI4OutMax=[]  SumDOutMin=[]  SumDOutMax=[]  DifferentiatorOutMin=[]  DifferentiatorOutMax=[]  FilterDiffOutCoefMin=[]  FilterDiffOutCoefMax=[]  ReciprocalOutMin=[]  ReciprocalOutMax=[]  SumDenOutMin=[]  SumDenOutMax=[]  SumNumOutMin=[]  SumNumOutMax=[]  DivideOutMin=[]  DivideOutMax=[]  UdiffTsProdOutMin=[]  UdiffTsProdOutMax=[]  NTsProdOutMin=[]  NTsProdOutMax=[]  UintegralTsProdOutMin=[]  UintegralTsProdOutMax=[]  UngainTsProdOutMin=[]  UngainTsProdOutMax=[]  IntegratorContinuousStateAttributes=''  IntegratorStateMustResolveToSignalObject=off  IntegratorRTWStateStorageClass=Auto  FilterContinuousStateAttributes=''  FilterStateMustResolveToSignalObject=off  FilterRTWStateStorageClass=Auto  ParallelPVariant=InternalParameters  IdealPVariant=Disabled  IVariant=Disabled  DVariant=InternalParameters  IntegratorVariant=Disabled  SatVariant=Disabled  AWVariant=Disabled  PCopyVariant=Disabled  TRVariant=Disabled  FdbkBlocksVariant=Forward  IdealPFdbkVariant=Disabled  SatFdbkVariant=Disabled  DerivativeFilterVariant=ForwardEulerFilter  NVariant=InternalParameters  NCopyVariant=Disabled  FilterICVariant=InternalICsFilter  IntegratorICVariant=Disabled  ExternalResetVariant=Disabled  TRSumVariant=Passthrough  SumFdbkVariant=Disabled  SumVariant=Sum_PD  TsampFilterVariant=InternalTs  TsampNgainVariant=Passthrough  TsampIntegralVariant=Disabled_SignalSpec  ExternalSaturationOutDataTypeStr=Inherit: Same as second input
  Discrete PID Controller3 : pid_lib/PID Controller  Controller=PD  Form=Parallel  TimeDomain=Discrete-time  UseExternalTs=off  SampleTime=T  IntegratorMethod=Forward Euler  FilterMethod=Forward Euler  ControllerParametersSource=internal  P=0.0348354109151771  I=Ki  D=1.99510127130573  UseFilter=on  N=145.233498095858  TunerSelectOption=Transfer Function Based (PID Tuner App)  InitialConditionSource=internal  InitialConditionForIntegrator=0  InitialConditionForFilter=0  DifferentiatorICPrevScaledInput=0  ExternalReset=none  TrackingMode=off  Kt=1  LimitOutput=off  SatLimitsSource=internal  UpperSaturationLimit=inf  LowerSaturationLimit=-inf  LinearizeAsGain=off  AntiWindupMode=none  Kb=1  POutMin=[]  POutMax=[]  IOutMin=[]  IOutMax=[]  DOutMin=[]  DOutMax=[]  NOutMin=[]  NOutMax=[]  SumOutMin=[]  SumOutMax=[]  SaturationOutMin=[]  SaturationOutMax=[]  PParamMin=[]  PParamMax=[]  IParamMin=[]  IParamMax=[]  DParamMin=[]  DParamMax=[]  NParamMin=[]  NParamMax=[]  KbParamMin=[]  KbParamMax=[]  KtParamMin=[]  KtParamMax=[]  KbOutMin=[]  KbOutMax=[]  KtOutMin=[]  KtOutMax=[]  IntegratorOutMin=[]  IntegratorOutMax=[]  FilterOutMin=[]  FilterOutMax=[]  SumI1OutMin=[]  SumI1OutMax=[]  SumI2OutMin=[]  SumI2OutMax=[]  SumI3OutMin=[]  SumI3OutMax=[]  SumI4OutMin=[]  SumI4OutMax=[]  SumDOutMin=[]  SumDOutMax=[]  DifferentiatorOutMin=[]  DifferentiatorOutMax=[]  FilterDiffOutCoefMin=[]  FilterDiffOutCoefMax=[]  ReciprocalOutMin=[]  ReciprocalOutMax=[]  SumDenOutMin=[]  SumDenOutMax=[]  SumNumOutMin=[]  SumNumOutMax=[]  DivideOutMin=[]  DivideOutMax=[]  UdiffTsProdOutMin=[]  UdiffTsProdOutMax=[]  NTsProdOutMin=[]  NTsProdOutMax=[]  UintegralTsProdOutMin=[]  UintegralTsProdOutMax=[]  UngainTsProdOutMin=[]  UngainTsProdOutMax=[]  IntegratorContinuousStateAttributes=''  IntegratorStateMustResolveToSignalObject=off  IntegratorRTWStateStorageClass=Auto  FilterContinuousStateAttributes=''  FilterStateMustResolveToSignalObject=off  FilterRTWStateStorageClass=Auto  ParallelPVariant=InternalParameters  IdealPVariant=Disabled  IVariant=Disabled  DVariant=InternalParameters  IntegratorVariant=Disabled  SatVariant=Disabled  AWVariant=Disabled  PCopyVariant=Disabled  TRVariant=Disabled  FdbkBlocksVariant=Forward  IdealPFdbkVariant=Disabled  SatFdbkVariant=Disabled  DerivativeFilterVariant=ForwardEulerFilter  NVariant=InternalParameters  NCopyVariant=Disabled  FilterICVariant=InternalICsFilter  IntegratorICVariant=Disabled  ExternalResetVariant=Disabled  TRSumVariant=Passthrough  SumFdbkVariant=Disabled  SumVariant=Sum_PD  TsampFilterVariant=InternalTs  TsampNgainVariant=Passthrough  TsampIntegralVariant=Disabled_SignalSpec  ExternalSaturationOutDataTypeStr=Inherit: Same as second input
  Mux : Mux
  w : Outport
  wires:
  e/1 -> Demux/1
  Discrete PID Controller2/1 -> Mux/3
  Demux/1 -> Discrete PID Controller/1
  Demux/3 -> Discrete PID Controller2/1
  Discrete PID Controller1/1 -> Mux/2
  Demux/2 -> Discrete PID Controller1/1
  Discrete PID Controller/1 -> Mux/1
  Mux/1 -> w/1
  Demux/4 -> Discrete PID Controller3/1
  Discrete PID Controller3/1 -> Mux/4

== system feedbackLinearizationMambo/Controller2/PD Magalhães ==
  e : Inport
  Demux1 : Demux  Outputs=3
  Discrete PID Controller3 : pid_lib/PID Controller  Controller=PD  Form=Parallel  TimeDomain=Discrete-time  UseExternalTs=off  SampleTime=T  IntegratorMethod=Forward Euler  FilterMethod=Forward Euler  ControllerParametersSource=internal  P=0.0004  I=Ki  D=0.0075  UseFilter=off  N=100  TunerSelectOption=Transfer Function Based (PID Tuner App)  InitialConditionSource=internal  InitialConditionForIntegrator=0  InitialConditionForFilter=0  DifferentiatorICPrevScaledInput=0  ExternalReset=none  TrackingMode=off  Kt=1  LimitOutput=off  SatLimitsSource=internal  UpperSaturationLimit=inf  LowerSaturationLimit=-inf  LinearizeAsGain=off  AntiWindupMode=none  Kb=1  POutMin=[]  POutMax=[]  IOutMin=[]  IOutMax=[]  DOutMin=[]  DOutMax=[]  NOutMin=[]  NOutMax=[]  SumOutMin=[]  SumOutMax=[]  SaturationOutMin=[]  SaturationOutMax=[]  PParamMin=[]  PParamMax=[]  IParamMin=[]  IParamMax=[]  DParamMin=[]  DParamMax=[]  NParamMin=[]  NParamMax=[]  KbParamMin=[]  KbParamMax=[]  KtParamMin=[]  KtParamMax=[]  KbOutMin=[]  KbOutMax=[]  KtOutMin=[]  KtOutMax=[]  IntegratorOutMin=[]  IntegratorOutMax=[]  FilterOutMin=[]  FilterOutMax=[]  SumI1OutMin=[]  SumI1OutMax=[]  SumI2OutMin=[]  SumI2OutMax=[]  SumI3OutMin=[]  SumI3OutMax=[]  SumI4OutMin=[]  SumI4OutMax=[]  SumDOutMin=[]  SumDOutMax=[]  DifferentiatorOutMin=[]  DifferentiatorOutMax=[]  FilterDiffOutCoefMin=[]  FilterDiffOutCoefMax=[]  ReciprocalOutMin=[]  ReciprocalOutMax=[]  SumDenOutMin=[]  SumDenOutMax=[]  SumNumOutMin=[]  SumNumOutMax=[]  DivideOutMin=[]  DivideOutMax=[]  UdiffTsProdOutMin=[]  UdiffTsProdOutMax=[]  NTsProdOutMin=[]  NTsProdOutMax=[]  UintegralTsProdOutMin=[]  UintegralTsProdOutMax=[]  UngainTsProdOutMin=[]  UngainTsProdOutMax=[]  IntegratorContinuousStateAttributes=''  IntegratorStateMustResolveToSignalObject=off  IntegratorRTWStateStorageClass=Auto  FilterContinuousStateAttributes=''  FilterStateMustResolveToSignalObject=off  FilterRTWStateStorageClass=Auto  ParallelPVariant=InternalParameters  IdealPVariant=Disabled  IVariant=Disabled  DVariant=InternalParameters  IntegratorVariant=Disabled  SatVariant=Disabled  AWVariant=Disabled  PCopyVariant=Disabled  TRVariant=Disabled  FdbkBlocksVariant=Forward  IdealPFdbkVariant=Disabled  SatFdbkVariant=Disabled  DerivativeFilterVariant=Differentiator  NVariant=Passthrough  NCopyVariant=Disabled_SignalSpec  FilterICVariant=InternalICsDifferentiator  IntegratorICVariant=Disabled  ExternalResetVariant=Disabled  TRSumVariant=Passthrough  SumFdbkVariant=Disabled  SumVariant=Sum_PD  TsampFilterVariant=InternalTs  TsampNgainVariant=Passthrough  TsampIntegralVariant=Disabled_SignalSpec  ExternalSaturationOutDataTypeStr=Inherit: Same as second input
  Discrete PID Controller4 : pid_lib/PID Controller  Controller=PD  Form=Parallel  TimeDomain=Discrete-time  UseExternalTs=off  SampleTime=T  IntegratorMethod=Forward Euler  FilterMethod=Forward Euler  ControllerParametersSource=internal  P=0.00025  I=Ki  D=0.0060  UseFilter=off  N=100  TunerSelectOption=Transfer Function Based (PID Tuner App)  InitialConditionSource=internal  InitialConditionForIntegrator=0  InitialConditionForFilter=0  DifferentiatorICPrevScaledInput=0  ExternalReset=none  TrackingMode=off  Kt=1  LimitOutput=off  SatLimitsSource=internal  UpperSaturationLimit=inf  LowerSaturationLimit=-inf  LinearizeAsGain=off  AntiWindupMode=none  Kb=1  POutMin=[]  POutMax=[]  IOutMin=[]  IOutMax=[]  DOutMin=[]  DOutMax=[]  NOutMin=[]  NOutMax=[]  SumOutMin=[]  SumOutMax=[]  SaturationOutMin=[]  SaturationOutMax=[]  PParamMin=[]  PParamMax=[]  IParamMin=[]  IParamMax=[]  DParamMin=[]  DParamMax=[]  NParamMin=[]  NParamMax=[]  KbParamMin=[]  KbParamMax=[]  KtParamMin=[]  KtParamMax=[]  KbOutMin=[]  KbOutMax=[]  KtOutMin=[]  KtOutMax=[]  IntegratorOutMin=[]  IntegratorOutMax=[]  FilterOutMin=[]  FilterOutMax=[]  SumI1OutMin=[]  SumI1OutMax=[]  SumI2OutMin=[]  SumI2OutMax=[]  SumI3OutMin=[]  SumI3OutMax=[]  SumI4OutMin=[]  SumI4OutMax=[]  SumDOutMin=[]  SumDOutMax=[]  DifferentiatorOutMin=[]  DifferentiatorOutMax=[]  FilterDiffOutCoefMin=[]  FilterDiffOutCoefMax=[]  ReciprocalOutMin=[]  ReciprocalOutMax=[]  SumDenOutMin=[]  SumDenOutMax=[]  SumNumOutMin=[]  SumNumOutMax=[]  DivideOutMin=[]  DivideOutMax=[]  UdiffTsProdOutMin=[]  UdiffTsProdOutMax=[]  NTsProdOutMin=[]  NTsProdOutMax=[]  UintegralTsProdOutMin=[]  UintegralTsProdOutMax=[]  UngainTsProdOutMin=[]  UngainTsProdOutMax=[]  IntegratorContinuousStateAttributes=''  IntegratorStateMustResolveToSignalObject=off  IntegratorRTWStateStorageClass=Auto  FilterContinuousStateAttributes=''  FilterStateMustResolveToSignalObject=off  FilterRTWStateStorageClass=Auto  ParallelPVariant=InternalParameters  IdealPVariant=Disabled  IVariant=Disabled  DVariant=InternalParameters  IntegratorVariant=Disabled  SatVariant=Disabled  AWVariant=Disabled  PCopyVariant=Disabled  TRVariant=Disabled  FdbkBlocksVariant=Forward  IdealPFdbkVariant=Disabled  SatFdbkVariant=Disabled  DerivativeFilterVariant=Differentiator  NVariant=Passthrough  NCopyVariant=Disabled_SignalSpec  FilterICVariant=InternalICsDifferentiator  IntegratorICVariant=Disabled  ExternalResetVariant=Disabled  TRSumVariant=Passthrough  SumFdbkVariant=Disabled  SumVariant=Sum_PD  TsampFilterVariant=InternalTs  TsampNgainVariant=Passthrough  TsampIntegralVariant=Disabled_SignalSpec  ExternalSaturationOutDataTypeStr=Inherit: Same as second input
  Discrete PID Controller5 : pid_lib/PID Controller  Controller=PD  Form=Parallel  TimeDomain=Discrete-time  UseExternalTs=off  SampleTime=T  IntegratorMethod=Forward Euler  FilterMethod=Forward Euler  ControllerParametersSource=internal  P=2e-05  I=Ki  D=0.00035  UseFilter=off  N=100  TunerSelectOption=Transfer Function Based (PID Tuner App)  InitialConditionSource=internal  InitialConditionForIntegrator=0  InitialConditionForFilter=0  DifferentiatorICPrevScaledInput=0  ExternalReset=none  TrackingMode=off  Kt=1  LimitOutput=off  SatLimitsSource=internal  UpperSaturationLimit=inf  LowerSaturationLimit=-inf  LinearizeAsGain=off  AntiWindupMode=none  Kb=1  POutMin=[]  POutMax=[]  IOutMin=[]  IOutMax=[]  DOutMin=[]  DOutMax=[]  NOutMin=[]  NOutMax=[]  SumOutMin=[]  SumOutMax=[]  SaturationOutMin=[]  SaturationOutMax=[]  PParamMin=[]  PParamMax=[]  IParamMin=[]  IParamMax=[]  DParamMin=[]  DParamMax=[]  NParamMin=[]  NParamMax=[]  KbParamMin=[]  KbParamMax=[]  KtParamMin=[]  KtParamMax=[]  KbOutMin=[]  KbOutMax=[]  KtOutMin=[]  KtOutMax=[]  IntegratorOutMin=[]  IntegratorOutMax=[]  FilterOutMin=[]  FilterOutMax=[]  SumI1OutMin=[]  SumI1OutMax=[]  SumI2OutMin=[]  SumI2OutMax=[]  SumI3OutMin=[]  SumI3OutMax=[]  SumI4OutMin=[]  SumI4OutMax=[]  SumDOutMin=[]  SumDOutMax=[]  DifferentiatorOutMin=[]  DifferentiatorOutMax=[]  FilterDiffOutCoefMin=[]  FilterDiffOutCoefMax=[]  ReciprocalOutMin=[]  ReciprocalOutMax=[]  SumDenOutMin=[]  SumDenOutMax=[]  SumNumOutMin=[]  SumNumOutMax=[]  DivideOutMin=[]  DivideOutMax=[]  UdiffTsProdOutMin=[]  UdiffTsProdOutMax=[]  NTsProdOutMin=[]  NTsProdOutMax=[]  UintegralTsProdOutMin=[]  UintegralTsProdOutMax=[]  UngainTsProdOutMin=[]  UngainTsProdOutMax=[]  IntegratorContinuousStateAttributes=''  IntegratorStateMustResolveToSignalObject=off  IntegratorRTWStateStorageClass=Auto  FilterContinuousStateAttributes=''  FilterStateMustResolveToSignalObject=off  FilterRTWStateStorageClass=Auto  ParallelPVariant=InternalParameters  IdealPVariant=Disabled  IVariant=Disabled  DVariant=InternalParameters  IntegratorVariant=Disabled  SatVariant=Disabled  AWVariant=Disabled  PCopyVariant=Disabled  TRVariant=Disabled  FdbkBlocksVariant=Forward  IdealPFdbkVariant=Disabled  SatFdbkVariant=Disabled  DerivativeFilterVariant=Differentiator  NVariant=Passthrough  NCopyVariant=Disabled_SignalSpec  FilterICVariant=InternalICsDifferentiator  IntegratorICVariant=Disabled  ExternalResetVariant=Disabled  TRSumVariant=Passthrough  SumFdbkVariant=Disabled  SumVariant=Sum_PD  TsampFilterVariant=InternalTs  TsampNgainVariant=Passthrough  TsampIntegralVariant=Disabled_SignalSpec  ExternalSaturationOutDataTypeStr=Inherit: Same as second input
  Mux1 : Mux  Inputs=3
  w : Outport
  wires:
  e/1 -> Demux1/1
  Discrete PID Controller3/1 -> Mux1/1
  Demux1/1 -> Discrete PID Controller3/1
  Demux1/3 -> Discrete PID Controller5/1
  Discrete PID Controller4/1 -> Mux1/2
  Discrete PID Controller5/1 -> Mux1/3
  Mux1/1 -> w/1
  Demux1/2 -> Discrete PID Controller4/1
